simulink model "Gemelo_Digital_RT_5_8_sinc_dig_real"  (R2025a)
settings: Solver=ode4  StartTime=0.0  StopTime=15  FixedStep=0.002  RelTol=1e-3  EnableMultiTasking=on
PreLoadFcn:
  | d=fileparts(get_param('Gemelo_Digital_RT_5_8_sinc_dig_real','FileName')); while ~isempty(d)&&~isfile(fullfile(d,'setup_paths.m')), n=fileparts(d); if strcmp(n,d),break;end; d=n; end; if isfile(fullfile(d,'setup_paths.m')), addpath(d); setup_paths; end
  | setup_swingup_quanser; Ensamblaje_pendulo_furuta_multibody_v4_DataFile;
InitFcn:
  | setup_swingup_quanser; Ensamblaje_pendulo_furuta_multibody_v4_DataFile;
undefined symbols (not defined in the file): alpha, alpha_m, g, HIL, Jp_cm, Ksync_tau, kt, l, mp, mr, p, qc_get_step_size, r, Rm, theta, theta_m, Vm, x_m, xhat
libraries: fl_lib x7, nesl_utility x7, simulink x5, quarc_library x4, sm_lib x2, ee_lib x1
settings Model: ExtModeTrigDuration=10000  Creator=sebas  LastModifiedBy=sebas
settings SolverCC: AlgebraicLoopSolver=TrustRegion  PositivePriorityOrder=on
settings DataIOCC: ReturnWorkspaceOutputs=off
settings DebuggingCC: UnconnectedInputMsg=warning  UnconnectedOutputMsg=warning  UnconnectedLineMsg=warning  ArithmeticOperatorsInVariantConditions=warning
settings ModelReferenceCC: EnableRefExpFcnMdlSchedulingChecks=on
settings SFSimCC: SimUseLocalCustomCode=off  CustomCodeUndefinedFunction=UseInterfaceOnly
settings RTWCC: SystemTargetFile=quarc_win64.tlc  TemplateMakefile=quarc_default_tmf  RTWUseLocalCustomCode=off  Toolchain=QUARC win64 | nmake (64-bit Windows)  BuildConfiguration=Faster Runs  GPUComputeCapability=3.5  Description=QUARC Win64 Target Using Toolchain
settings CodeAppCC: StateflowObjectComments=on
settings STFCustomTargetCC: SystemTargetFile=quarc_win64.tlc  TargetLangStandard=C99 (ISO)  MultiwordLength=2048.0  DynamicStringBufferSize=256.0  ConcurrentExecutionCompliant=on  UseToolchainInfoCompliant=on
settings ConfigComp: CovMetricSettings=dswe

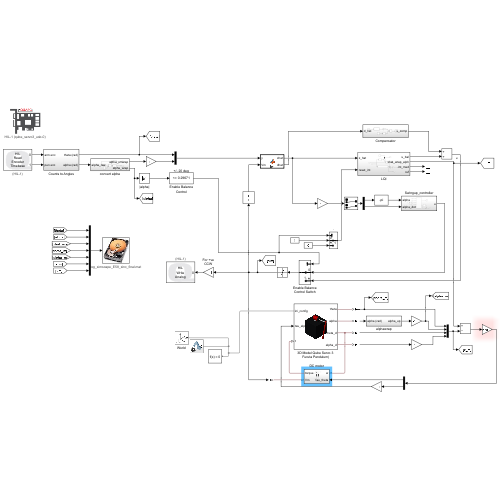
[thumbnail: Simulink's stored preview of the top-level diagram]
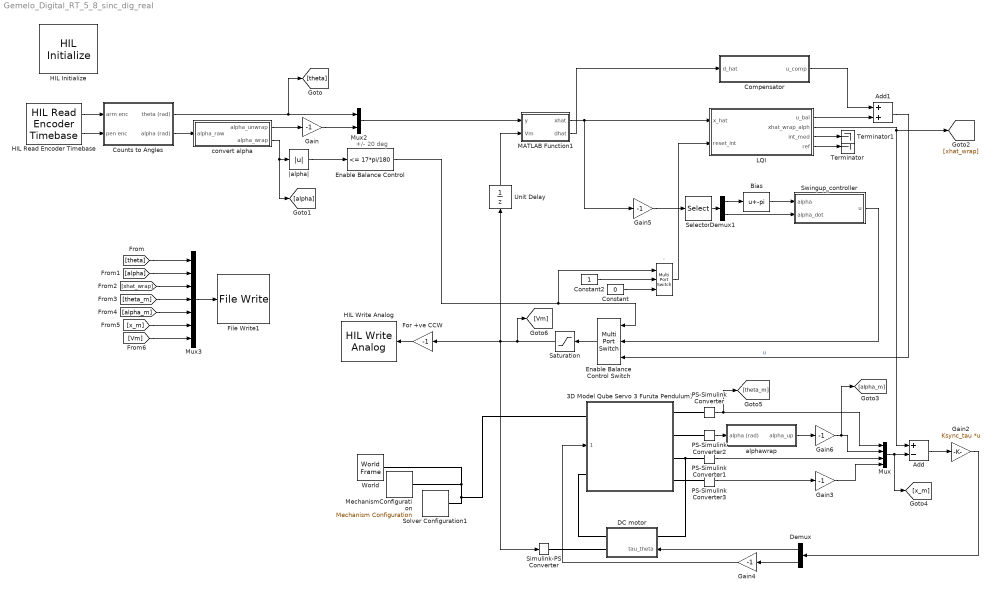
== system Gemelo_Digital_RT_5_8_sinc_dig_real ==
  note: +/- 20 deg
  . : MultiPortSwitch  DataPortOrder=Zero-based contiguous  Inputs=2  zeroidx=on  SaturateOnIntegerOverflow=off  InputSameDT=off
  3D Model Qube Servo 3 Furuta Pendulum) : Subsystem  ReferencedSubsystem=Model3d_Furuta_Pendulum
      settings: PortSchema="{\"entries\":[{\"content\":{\"sides\":[{\"content\":{\"connectorIds\":[\"LConn1\",\"In1\",\"RConn1\"]},\"type\":\"ConnectorPlacement.EquallySpacedRectSide\",\"uuid\":\"212e22e8-83aa-4288-bac8-5ec5012ee4e1\"},{\"content\":{\"connectorIds\":[\"RConn2\",\"RConn3\",\"RConn4\",\"RConn5\"],\"side\":\"RIGHT\"},\"type\":\"ConnectorPlacement.EquallySpacedRectSide\",\"uuid\":\"3ce73576-5c91-4b8f-99f3-bf7d5d6df258\"},{\"content\":{\"side\":\"TOP\"},\"type\":\"ConnectorPlacement.EquallySpacedRectSide\",\"uuid\":\"0c3f09e1-5576-45f6-bf17-671c1b7b7e25\"}]},\"type\":\"ConnectorPlacement.EquallySpacedConnector\",\"uuid\":\"8a7c1845-9713-4869-bdf4-33668feaed10\"}],\"packageUris\":[\"http://schema.mathworks.com/mf0/Connector/R2020b\"],\"version\":\"1.0\"}"
  Add : Sum  Inputs=+-
  Add1 : Sum
  Bias : Bias  Bias=-pi  SaturateOnIntegerOverflow=off
  Compensator : Subsystem
  Constant : Constant  Value=0
  Constant2 : Constant
  Counts to Angles : Subsystem
  DC motor : Subsystem
      settings: PortSchema="{\"entries\":[{\"content\":{\"sides\":[{\"content\":{\"connectorIds\":[\"LConn1\",\"In1\"]},\"type\":\"ConnectorPlacement.EquallySpacedRectSide\",\"uuid\":\"69bd88ca-8c2a-4f56-9568-a6ac34231cb3\"},{\"content\":{\"connectorIds\":[\"RConn1\",\"RConn2\"],\"side\":\"RIGHT\"},\"type\":\"ConnectorPlacement.EquallySpacedRectSide\",\"uuid\":\"19dd9353-83e6-4777-a984-67df33566e37\"},{\"content\":{\"side\":\"TOP\"},\"type\":\"ConnectorPlacement.EquallySpacedRectSide\",\"uuid\":\"45c5d2e2-678e-4947-ac23-f07febb6517c\"}]},\"type\":\"ConnectorPlacement.EquallySpacedConnector\",\"uuid\":\"c676389f-ef6f-4d18-b05a-27f295148147\"}],\"packageUris\":[\"http://schema.mathworks.com/mf0/Connector/R2020b\"],\"version\":\"1.0\"}"
  Demux : Demux  Outputs=2
  Demux1 : Demux  Outputs=2
  Enable Balance Control : simulink/Logic and Bit Operations/Compare To Constant  relop=<=  const=17*pi/180  OutDataTypeStr=boolean  ZeroCross=off
  Enable Balance Control Switch : MultiPortSwitch  DataPortOrder=Zero-based contiguous  Inputs=2  zeroidx=on  SaturateOnIntegerOverflow=off  InputSameDT=off
  File Write1 : quarc_library/Sinks/To Target/File Write  source=Specify via dialog (do not evaluate)  file_name=log_simscape_E58_sinc_final.mat  variable_name=theta,alpha,xhat,theta_m,alpha_m,x_m,Vm  decimation=1  sample_time=-1  file_format=MAT-file v.4  options=No header or footer  append=off  encoding=Default  bitrate=0
      settings: AttributesFormatString=%<file_name>  SourceProductName=QUARC Targets
  For +ve CCW : Gain  Gain=-1
  Gain{,3..6} (5 alike) : Gain  Gain=-1
  Gain2 : Gain  Gain=Ksync_tau  Multiplication=Matrix(K*u)
  HIL Initialize : quarc_library/Data Acquisition/Generic/Configuration/HIL Initialize  object_name=HIL-1  board_type=qube_servo3_usb  board_number=0  board_options=deadband_compensation=0.3;pwm_en=0;enc0_velocity=3.0;enc1_velocity=3.0;min_diode_compensation=0.3;max_diode_compensation=1.5;  exclusive=off  active=on  hardware_clocks=[0]  clock_modes=[]  initial_clock_frequencies=[]  set_clock_params_at_start=off  set_clock_params_at_switch_in=off  set_clock_frequencies_at_start=off  set_clock_frequencies_at_switch_in=off  analog_input_channels=[0]  analog_input_configurations=[]  analog_input_maximums=3  analog_input_minimums=-3  set_analog_input_params_at_start=off  set_analog_input_params_at_switch_in=off  analog_output_channels=[0]  analog_output_maximums=15  analog_output_minimums=-15  initial_analog_outputs=[0]  final_analog_outputs=[0]  watchdog_analog_outputs=0  set_analog_output_params_at_start=off  set_analog_output_params_at_switch_in=off  set_analog_outputs_at_start=on  set_analog_outputs_at_switch_in=off  set_analog_outputs_at_terminate=on  set_analog_outputs_at_switch_out=off  set_analog_outputs_on_watchdog=on  digital_input_channels=[]  digital_output_channels=[0]  digital_output_configuration=[]  initial_digital_outputs=[1]  final_digital_outputs=[0]  watchdog_digital_outputs=[0]  set_digital_output_params_at_start=off  set_digital_output_params_at_switch_in=off  set_digital_outputs_at_start=on  set_digital_outputs_at_switch_in=off  set_digital_outputs_at_terminate=on  set_digital_outputs_at_switch_out=off  set_digital_outputs_on_watchdog=on  encoder_channels=[0:1]  quadrature=[4]  encoder_filter_frequency=[]  initial_encoder_counts=[0]  set_encoder_params_at_start=off  set_encoder_params_at_switch_in=off  set_encoder_counts_at_start=on  set_encoder_counts_at_switch_in=off  pwm_channels=[]  pwm_modes=[0]  pwm_frequency=23195  pwm_configuration=[1]  pwm_alignment=[0]  pwm_polarity=[1]  pwm_leading_deadband=[0]  pwm_trailing_deadband=[0]  initial_pwm_outputs=[0]  final_pwm_outputs=[0]  watchdog_pwm_outputs=[]  set_pwm_params_at_start=off  set_pwm_params_at_switch_in=off  set_pwm_outputs_at_start=off  set_pwm_outputs_at_switch_in=off  set_pwm_outputs_at_terminate=off  set_pwm_outputs_at_switch_out=off  set_pwm_outputs_on_watchdog=off  other_output_channels=[11000:11002]  initial_other_outputs=[0 1 0]  final_other_outputs=[1 0 0]  watchdog_other_outputs=[0 0 1]  set_other_outputs_at_start=on  set_other_outputs_at_switch_in=off  set_other_outputs_at_terminate=on  set_other_outputs_at_switch_out=off  set_other_outputs_on_watchdog=on
  HIL Read Encoder Timebase : quarc_library/Data Acquisition/Generic/Timebases/HIL Read Encoder Timebase  object_name=HIL-1  clock=0  channels=[0:1]  active=on  vector_output=off  data_type_mode=Inherit via back propagation  data_type=double  overflow_mode=Error on overflow  samples_in_buffer=max(ceil(1/qc_get_step_size), 1)
  HIL Write Analog : quarc_library/Data Acquisition/Generic/Immediate I//O/HIL Write Analog  object_name=HIL-1  channels=[0]  sample_time=-1  active=off  vector_input=off
  LQI : Subsystem
  MATLAB Function1 : MATLAB Function  TreatAsAtomicUnit=on
  MechanismConfiguration : sm_lib/Utilities/Mechanism Configuration  UniformGravity=Constant  GravityVector=[0 -9.7807 0]  GravityVectorUnits=m/s^2  LinearizationDelta=0.001  JointModeTransitionNonlinearIterations=2
  Mux : Mux
  Mux2 : Mux  Inputs=2
  Mux3 : Mux  Inputs=7
  PS-Simulink Converter{,1..3} (4 alike) : nesl_utility/PS-Simulink Converter  PhysicalDomain=network_engine_domain  SubClassName=ps_output  LeftPortType=input  RightPortType=output  PseudoPeriodic=off  Frequencies=[]  VectorFormat=inherit  Unit=inherit  AffineConversion=off
  Saturation : Saturate  UpperLimit=10  LowerLimit=-10
  Selector : Selector  InputPortWidth=4  IndexOptions=Index vector (dialog)  Indices=[2 4]  OutputSizes=1
  Simulink-PS Converter : nesl_utility/Simulink-PS Converter  PhysicalDomain=network_engine_domain  SubClassName=ps_input  LeftPortType=input  RightPortType=output  PseudoPeriodic=off  Frequencies=[]  NoiseDistribution=none  NoiseParameters=[]  Unit=1  AffineConversion=off  FilteringAndDerivatives=filter  SimscapeFilterOrder=1  InputFilterTimeConstant=0.001  UdotUserProvided=0
  Solver Configuration1 : nesl_utility/Solver Configuration  PhysicalDomain=network_engine_domain  SubClassName=solver  LeftPortType=input  RightPortType=generic  Tones=[]  Harmonics=[]  SimulateNoise=off  Profile=off  UseLocalSampling=off  EnableSwitchedLinearOptims=on  FrequencyDomain=off  UseCCode=off  RelTol=0.001  AbsTol=0.001  MinStep=1e-09  ToWorkspace=off  RevertToSquareIcSolve=off  NumHomotopyIterations=100  PhasorMode=off  PhasorModeNumHarmonics=1  ConsistencySolver=NEWTON_XTOL_AFTER_FTOL  IndexReductionMethod=DerivativeReplacement  DoDC=off  ResidualTolerance=1e-09  ConsistencyTolSource=GLOBAL  ConsistencyAbsTol=0.001  ConsistencyRelTol=0.001  ConsistencyTolFactor=1e-9  UseLocalSolver=on  LocalSolverChoice=NE_BACKWARD_EULER_ADVANCER  ResolveIndetEquations=on  FunctionEvalNumThread=1  LocalSolverSampleTime=0.002  DoFixedCost=on  MaxNonlinIter=5  MaxModeIter=2  ComputeImpulses=on  ImpulseIterations=2  LinearAlgebra=auto  LinearAlgebraNumThread=0  EquationFormulation=NE_TIME_EF  DelaysMemoryBudget=1024  AutomaticFiltering=on  FilteringTimeConstant=0.001  PartitionStorageMethod=AS_NEEDED  PartitionMemoryBudget=1024  PartitionMethod=ROBUST  MultibodyUseLocalSolver=off  MultibodyLocalSolverChoice=ODE1  MultibodyLocalSolverSampleTime=0.002
  Swingup_controller : Subsystem
  Terminator : Terminator
  Terminator1 : Terminator
  Unit Delay : UnitDelay  SampleTime=-1  HasFrameUpgradeWarning=on
  World : sm_lib/Frames and Transforms/World Frame
  alphawrap : Subsystem
  convert alpha : Subsystem
  |alpha| : Abs  SaturateOnIntegerOverflow=off
  wires:
  Gain4/1 -> 3D Model Qube Servo 3 Furuta Pendulum)/1
  PS-Simulink Converter/1 -> [theta_m], Mux/1
  alphawrap/1(alpha_up) -> Gain6/1
  PS-Simulink Converter3/1 -> Gain3/1
  Gain3/1 -> Mux/4
  PS-Simulink Converter1/1 -> Mux/3
  Gain2/1 -> Demux/1
  LQI/2(xhat_wrap_alph) -> [xhat_wrap], Add/1
  Add/1 -> Gain2/1
  Demux/1 -> DC motor/1(tau_theta)
  Demux/2 -> Gain4/1
  Mux/1 -> [x_m], Add/2
  Counts to Angles/1(theta (rad)) -> [theta], Mux2/1
  HIL Read Encoder Timebase/2 -> Counts to Angles/2(pen enc)
  HIL Read Encoder Timebase/1 -> Counts to Angles/1(arm enc)
  Saturation/1 -> [Vm], Simulink-PS Converter/1, For +ve CCW/1, Unit Delay/1
  MATLAB Function1/2(dhat) -> Compensator/1(d_hat)
  Mux3/1 -> File Write1/1
  MATLAB Function1/1(xhat) -> Gain5/1, LQI/1(x_hat)
  Swingup_controller/1(u) -> Enable Balance Control Switch/2
  LQI/1(u_bal) -> Add1/2
  Constant/1 -> ./3
  Counts to Angles/2(alpha (rad)) -> convert alpha/1(alpha_raw)
  Add1/1 -> Enable Balance Control Switch/3  "u"
  Demux1/2 -> Swingup_controller/2(alpha_dot)
  Constant2/1 -> ./2
  convert alpha/2(alpha_wrap) -> [alpha], |alpha|/1
  Gain5/1 -> Selector/1
  Selector/1 -> Demux1/1
  |alpha|/1 -> Enable Balance Control/1
  Demux1/1 -> Bias/1
  ./1 -> LQI/2(reset_int)
  Enable Balance Control Switch/1 -> Saturation/1
  convert alpha/1(alpha_unwrap) -> Gain/1
  Enable Balance Control/1 -> Enable Balance Control Switch/1, ./1
  For +ve CCW/1 -> HIL Write Analog/1
  Mux2/1 -> MATLAB Function1/1(y)
  Bias/1 -> Swingup_controller/1(alpha)
  Unit Delay/1 -> MATLAB Function1/2(Vm)
  Compensator/1(u_comp) -> Add1/1
  PS-Simulink Converter2/1 -> alphawrap/1(alpha (rad))
  Gain/1 -> Mux2/2
  Gain6/1 -> [alpha_m], Mux/2
  LQI/4(ref) -> Terminator/1
  LQI/3(int_med) -> Terminator1/1
  [theta] -> Mux3/1
  [alpha] -> Mux3/2
  [xhat_wrap] -> Mux3/3
  [theta_m] -> Mux3/4
  [alpha_m] -> Mux3/5
  [x_m] -> Mux3/6
  [Vm] -> Mux3/7
  connections:
  World/RConn1 -- MechanismConfiguration/RConn1 -- Solver Configuration1/RConn1 -- 3D Model Qube Servo 3 Furuta Pendulum)/LConn1
  Simulink-PS Converter/RConn1 -- DC motor/RConn2
  3D Model Qube Servo 3 Furuta Pendulum)/RConn2 -- PS-Simulink Converter/LConn1
  3D Model Qube Servo 3 Furuta Pendulum)/RConn3 -- PS-Simulink Converter2/LConn1
  3D Model Qube Servo 3 Furuta Pendulum)/RConn4 -- DC motor/LConn1 -- PS-Simulink Converter1/LConn1
  3D Model Qube Servo 3 Furuta Pendulum)/RConn5 -- PS-Simulink Converter3/LConn1
  DC motor/RConn1 -- 3D Model Qube Servo 3 Furuta Pendulum)/RConn1

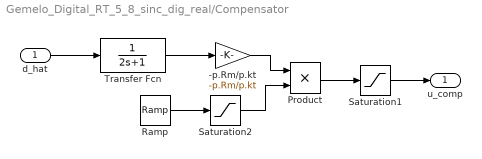
== system Gemelo_Digital_RT_5_8_sinc_dig_real/Compensator ==
  d_hat : Inport
  -p.Rm/p.kt : Gain  Gain=-p.Rm/p.kt
  Product : Product
  Ramp : simulink/Sources/Ramp  slope=0.5  start=0  InitialOutput=0
  Saturation1 : Saturate  UpperLimit=2  LowerLimit=-2
  Saturation2 : Saturate  UpperLimit=1  LowerLimit=0
  Transfer Fcn : TransferFcn  Denominator=[2 1]
  u_comp : Outport
  wires:
  Saturation1/1 -> u_comp/1
  Transfer Fcn/1 -> -p.Rm/p.kt/1
  -p.Rm/p.kt/1 -> Product/1
  Saturation2/1 -> Product/2
  Ramp/1 -> Saturation2/1
  d_hat/1 -> Transfer Fcn/1
  Product/1 -> Saturation1/1

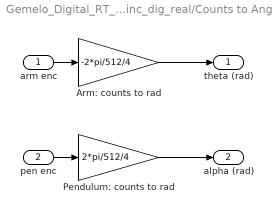
== system Gemelo_Digital_RT_5_8_sinc_dig_real/Counts to Angles ==
  arm enc : Inport
  pen enc : Inport  Port=2
  Arm: counts to rad : Gain  Gain=-2*pi/512/4
  Pendulum: counts to rad : Gain  Gain=2*pi/512/4
  theta (rad) : Outport  VectorParamsAs1DForOutWhenUnconnected=off
  alpha (rad) : Outport  Port=2  VectorParamsAs1DForOutWhenUnconnected=off
  wires:
  pen enc/1 -> Pendulum: counts to rad/1
  arm enc/1 -> Arm: counts to rad/1
  Arm: counts to rad/1 -> theta (rad)/1
  Pendulum: counts to rad/1 -> alpha (rad)/1

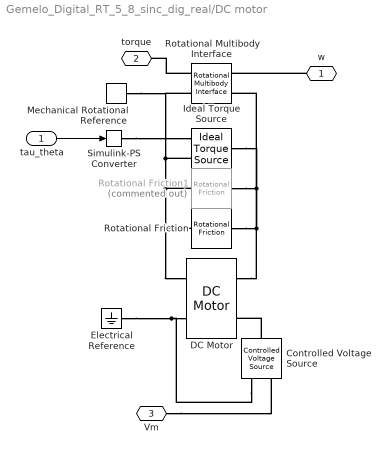
== system Gemelo_Digital_RT_5_8_sinc_dig_real/DC motor ==
  tau_theta : Inport
  Controlled Voltage Source : fl_lib/Electrical/Electrical Sources/Controlled Voltage Source
  DC Motor : ee_lib/Electromechanical/Brushed Motors/DC Motor  field_option=ee.enum.field_option.pm  Rf=100 Ohm  Lf=1 H  Laf=0.15 H  If0=0 A  parameterization=ee.enum.dcparam_option.circuit_param  Ra=7.5 Ohm  La=1.15e-3 H  emf_or_torque=ee.enum.emf_or_torque.kv  Kv=0.0422 V*s/rad  Ki=0.0422 N*m/A  T_stall=0.24e-3 N*m  w_max=5400 rpm  w_rated=4579 rpm  P_rated=9.8 W  V_rated=24 V  lam_param=ee.enum.lam_param.damping  i_noload=16 mA  V_i_noload=24 V  J=1.4e-6 kg*m^2  lam=1*4.8390e-6 N*m*s/rad  speed0=0 rpm  alpha=3.93e-3 1/K  Tmeas=25 degC  thermal_mass=100 J/K  initial_temperature=25 degC
  Electrical Reference : fl_lib/Electrical/Electrical Elements/Electrical Reference
  Ideal Torque Source : fl_lib/Mechanical/Mechanical Sources/Ideal Torque Source
  Mechanical Rotational Reference : fl_lib/Mechanical/Rotational Elements/Mechanical Rotational Reference
  Rotational Friction : fl_lib/Mechanical/Rotational Elements/Rotational Friction  brkwy_trq=1*2.910555e-05+1*4.081637e-05 N*m  brkwy_vel=1.082312e-02 rad/s  Col_trq=2.910555e-05 N*m  visc_coef=4.321929e-06 N*m*s/rad  w_specify=off  w_priority=None  w=0 rad/s  w_nominal_specify=off  w_nominal_value=1  w_nominal_unit=rad/s  t_specify=off  t_priority=None  t=0 N*m  t_nominal_specify=off  t_nominal_value=1  t_nominal_unit=N*m
  Rotational Friction1 : fl_lib/Mechanical/Rotational Elements/Rotational Friction  Commented=on  brkwy_trq=7.066e-04 N*m  brkwy_vel=0.1 rad/s  Col_trq=7.066e-09 N*m  visc_coef=0 N*m*s/rad  w_specify=off  w_priority=None  w=0 rad/s  w_nominal_specify=off  w_nominal_value=1  w_nominal_unit=rad/s  t_specify=off  t_priority=None  t=0 N*m  t_nominal_specify=off  t_nominal_value=1  t_nominal_unit=N*m
  Rotational Multibody Interface : fl_lib/Mechanical/Multibody Interfaces/Rotational Multibody Interface
  Simulink-PS Converter : nesl_utility/Simulink-PS Converter  PhysicalDomain=network_engine_domain  SubClassName=ps_input  LeftPortType=input  RightPortType=output  PseudoPeriodic=off  Frequencies=[]  NoiseDistribution=none  NoiseParameters=[]  Unit=1  AffineConversion=off  FilteringAndDerivatives=filter  SimscapeFilterOrder=1  InputFilterTimeConstant=0.001  UdotUserProvided=0
  w : PMIOPort  Side=Left
  torque : PMIOPort  Port=2  Side=Right
  Vm : PMIOPort  Port=3  Side=Right
  wires:
  tau_theta/1 -> Simulink-PS Converter/1
  connections:
  Rotational Friction/LConn1 -- Rotational Friction1/LConn1 -- Ideal Torque Source/LConn1 -- Rotational Multibody Interface/RConn2 -- DC Motor/LConn2
  Rotational Friction/RConn1 -- Ideal Torque Source/RConn2 -- Rotational Multibody Interface/LConn2 -- Mechanical Rotational Reference/LConn1 -- Rotational Friction1/RConn1 -- DC Motor/RConn2
  Vm/RConn1 -- Controlled Voltage Source/RConn1
  w/RConn1 -- Rotational Multibody Interface/RConn1
  DC Motor/RConn1 -- Electrical Reference/LConn1 -- Controlled Voltage Source/RConn2
  Controlled Voltage Source/LConn1 -- DC Motor/LConn1
  Rotational Multibody Interface/LConn1 -- torque/RConn1
  Simulink-PS Converter/RConn1 -- Ideal Torque Source/RConn1

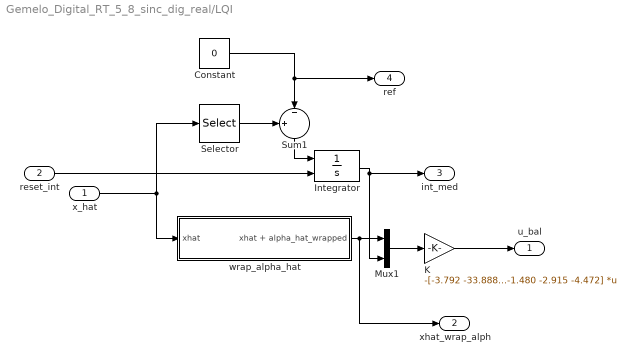
== system Gemelo_Digital_RT_5_8_sinc_dig_real/LQI ==
  x_hat : Inport
  reset_int : Inport  Port=2
  Constant : Constant  Value=0
  Integrator : Integrator  ExternalReset=level hold  LimitOutput=on  UpperSaturationLimit=2  LowerSaturationLimit=-2
  K : Gain  Gain=-[-3.792 -33.888 -1.480 -2.915 -4.472]  Multiplication=Matrix(K*u)
  Mux1 : Mux  Inputs=2
  Selector : Selector  InputPortWidth=4  IndexOptions=Index vector (dialog)  Indices=[1]  OutputSizes=1
  Sum1 : Sum  Inputs=+|-||
  wrap_alpha_hat : Subsystem
  u_bal : Outport
  xhat_wrap_alph : Outport  Port=2
  int_med : Outport  Port=3
  ref : Outport  Port=4
  wires:
  Integrator/1 -> int_med/1, Mux1/2
  Mux1/1 -> K/1
  Constant/1 -> ref/1, Sum1/2
  Sum1/1 -> Integrator/1
  Selector/1 -> Sum1/1
  K/1 -> u_bal/1
  reset_int/1 -> Integrator/2
  x_hat/1 -> wrap_alpha_hat/1(xhat), Selector/1
  wrap_alpha_hat/1(xhat + alpha_hat_wrapped) -> xhat_wrap_alph/1, Mux1/1

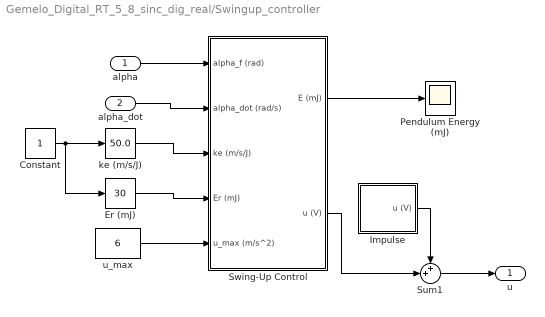
== system Gemelo_Digital_RT_5_8_sinc_dig_real/Swingup_controller ==
  alpha : Inport
  alpha_dot : Inport  Port=2
  Constant : Constant
  Er (mJ) : simulink/Math Operations/Slider Gain  gain=30  low=0  high=100
  Impulse : Subsystem
  Pendulum Energy (mJ) : Scope
      settings: ActiveDisplayYMinimum=-1.7076335355968837  ActiveDisplayYMaximum=4.1343640569805871  DataLoggingVariableName=ScopeData3
  Sum1 : Sum  Inputs=++|
  Swing-Up Control : Subsystem
  ke (m/s/J) : simulink/Math Operations/Slider Gain  gain=50.0  low=0  high=100
  u_max : Constant  Value=6
  u : Outport
  wires:
  alpha/1 -> Swing-Up Control/1(alpha_f (rad))
  Sum1/1 -> u/1
  u_max/1 -> Swing-Up Control/5(u_max (m/s^2))
  Impulse/1(u (V)) -> Sum1/1
  Swing-Up Control/1(E (mJ)) -> Pendulum Energy (mJ)/1
  Swing-Up Control/2(u (V)) -> Sum1/2
  ke (m/s/J)/1 -> Swing-Up Control/3(ke (m/s/J))
  Constant/1 -> Er (mJ)/1, ke (m/s/J)/1
  Er (mJ)/1 -> Swing-Up Control/4(Er (mJ))
  alpha_dot/1 -> Swing-Up Control/2(alpha_dot (rad/s))

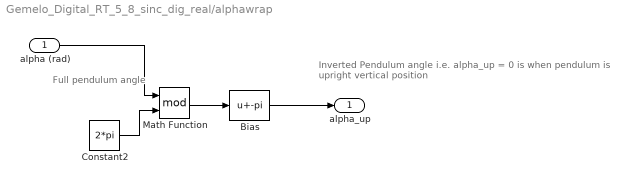
== system Gemelo_Digital_RT_5_8_sinc_dig_real/alphawrap ==
  note: Full pendulum angle
  note: Inverted Pendulum angle
      | i.e. alpha_up = 0 is when pendulum is upright vertical position
  alpha (rad) : Inport
  Bias : Bias  Bias=-pi  SaturateOnIntegerOverflow=off
  Constant2 : Constant  Value=2*pi
  Math Function : Math  Operator=mod  SignedPower=on
  alpha_up : Outport  VectorParamsAs1DForOutWhenUnconnected=off
  wires:
  Math Function/1 -> Bias/1
  Bias/1 -> alpha_up/1
  Constant2/1 -> Math Function/2
  alpha (rad)/1 -> Math Function/1

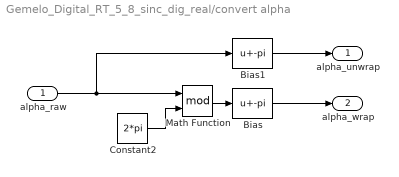
== system Gemelo_Digital_RT_5_8_sinc_dig_real/convert alpha ==
  alpha_raw : Inport
  Bias : Bias  Bias=-pi  SaturateOnIntegerOverflow=off
  Bias1 : Bias  Bias=-pi  SaturateOnIntegerOverflow=off
  Constant2 : Constant  Value=2*pi
  Math Function : Math  Operator=mod  SignedPower=on
  alpha_unwrap : Outport
  alpha_wrap : Outport  Port=2
  wires:
  Math Function/1 -> Bias/1
  Bias/1 -> alpha_wrap/1
  Constant2/1 -> Math Function/2
  alpha_raw/1 -> Bias1/1, Math Function/1
  Bias1/1 -> alpha_unwrap/1

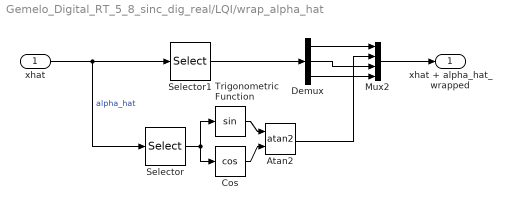
== system Gemelo_Digital_RT_5_8_sinc_dig_real/LQI/wrap_alpha_hat ==
  xhat : Inport
  Atan2 : Trigonometry  Operator=atan2
  Cos : Trigonometry  Operator=cos
  Demux : Demux  Outputs=3
  Mux2 : Mux
  Selector : Selector  InputPortWidth=4  IndexOptions=Index vector (dialog)  Indices=[2]  OutputSizes=1
  Selector1 : Selector  InputPortWidth=4  IndexOptions=Index vector (dialog)  Indices=[1 3 4]  OutputSizes=1
  Trigonometric Function : Trigonometry
  xhat + alpha_hat_wrapped : Outport
  wires:
  Selector/1 -> Cos/1, Trigonometric Function/1
  Mux2/1 -> xhat + alpha_hat_wrapped/1
  Cos/1 -> Atan2/2
  xhat/1 -> Selector/1, Selector1/1  "alpha_hat"
  Trigonometric Function/1 -> Atan2/1
  Demux/2 -> Mux2/3
  Selector1/1 -> Demux/1
  Demux/1 -> Mux2/1
  Demux/3 -> Mux2/4
  Atan2/1 -> Mux2/2

== system Gemelo_Digital_RT_5_8_sinc_dig_real/Swingup_controller/Impulse ==
  Impulse Amplitude : Gain  Gain=0.2
  Step : Step  SampleTime=0
  Step1 : Step  Time=1.1  After=-1  SampleTime=0
  Sum : Sum  Inputs=|++
  u (V) : Outport  VectorParamsAs1DForOutWhenUnconnected=off
  wires:
  Impulse Amplitude/1 -> u (V)/1
  Sum/1 -> Impulse Amplitude/1
  Step/1 -> Sum/1
  Step1/1 -> Sum/2

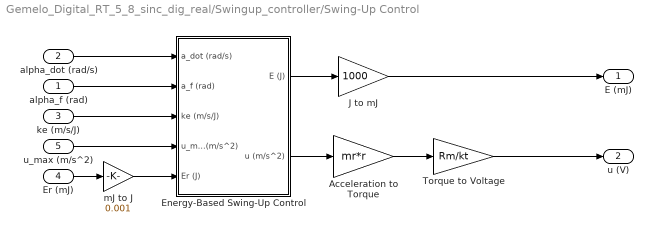
== system Gemelo_Digital_RT_5_8_sinc_dig_real/Swingup_controller/Swing-Up Control ==
  alpha_f (rad) : Inport
  alpha_dot (rad/s) : Inport  Port=2
  ke (m/s/J) : Inport  Port=3
  Er (mJ) : Inport  Port=4
  u_max (m/s^2) : Inport  Port=5
  Acceleration to Torque : Gain  Gain=mr*r
  Energy-Based Swing-Up Control : Subsystem
  J to mJ : Gain  Gain=1000
  Torque to Voltage : Gain  Gain=Rm/kt
  mJ to J : Gain  Gain=0.001
  E (mJ) : Outport  VectorParamsAs1DForOutWhenUnconnected=off
  u (V) : Outport  Port=2  VectorParamsAs1DForOutWhenUnconnected=off
  wires:
  mJ to J/1 -> Energy-Based Swing-Up Control/5(Er (J))
  alpha_dot (rad/s)/1 -> Energy-Based Swing-Up Control/1(a_dot (rad/s))
  Torque to Voltage/1 -> u (V)/1
  J to mJ/1 -> E (mJ)/1
  Er (mJ)/1 -> mJ to J/1
  Acceleration to Torque/1 -> Torque to Voltage/1
  u_max (m/s^2)/1 -> Energy-Based Swing-Up Control/4(u_max (m/s^2))
  ke (m/s/J)/1 -> Energy-Based Swing-Up Control/3(ke (m/s/J))
  alpha_f (rad)/1 -> Energy-Based Swing-Up Control/2(a_f (rad))
  Energy-Based Swing-Up Control/1(E (J)) -> J to mJ/1
  Energy-Based Swing-Up Control/2(u (m/s^2)) -> Acceleration to Torque/1

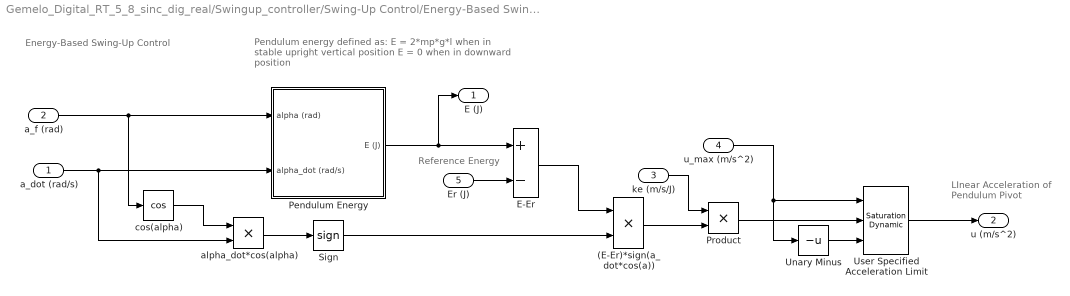
== system Gemelo_Digital_RT_5_8_sinc_dig_real/Swingup_controller/Swing-Up Control/Energy-Based Swing-Up Control ==
  note: Pendulum energy defined as:
      | E = 2*mp*g*l when in stable upright vertical position
      | E = 0 when in downward position
  note: Reference Energy
  note: LInear Acceleration of
      | Pendulum Pivot
  note: Energy-Based Swing-Up Control
  a_dot (rad/s) : Inport
  a_f (rad) : Inport  Port=2
  ke (m/s/J) : Inport  Port=3
  u_max (m/s^2) : Inport  Port=4
  Er (J) : Inport  Port=5
  (E-Er)*sign(a_dot*cos(a)) : Product  RndMeth=Zero
  E-Er : Sum  Inputs=+-
  Pendulum Energy : Subsystem
  Product : Product  RndMeth=Zero
  Sign : Signum
  Unary Minus : UnaryMinus
  User Specified Acceleration Limit : simulink/Discontinuities/Saturation Dynamic  OutMin=[]  OutMax=[]  OutDataTypeStr=Inherit: Same as second input  OutDataType=fixdt(1, 16)  OutScaling=2^-10  DoSatur=off
  alpha_dot*cos(alpha) : Product  RndMeth=Zero
  cos(alpha) : Trigonometry  Operator=cos
  E (J) : Outport  VectorParamsAs1DForOutWhenUnconnected=off
  u (m/s^2) : Outport  Port=2  VectorParamsAs1DForOutWhenUnconnected=off
  wires:
  User Specified Acceleration Limit/1 -> u (m/s^2)/1
  Unary Minus/1 -> User Specified Acceleration Limit/3
  u_max (m/s^2)/1 -> Unary Minus/1, User Specified Acceleration Limit/1
  Product/1 -> User Specified Acceleration Limit/2
  ke (m/s/J)/1 -> Product/1
  Er (J)/1 -> E-Er/2
  (E-Er)*sign(a_dot*cos(a))/1 -> Product/2
  a_dot (rad/s)/1 -> Pendulum Energy/2(alpha_dot (rad/s)), alpha_dot*cos(alpha)/2
  Pendulum Energy/1(E (J)) -> E-Er/1, E (J)/1
  E-Er/1 -> (E-Er)*sign(a_dot*cos(a))/1
  cos(alpha)/1 -> alpha_dot*cos(alpha)/1
  alpha_dot*cos(alpha)/1 -> Sign/1
  Sign/1 -> (E-Er)*sign(a_dot*cos(a))/2
  a_f (rad)/1 -> cos(alpha)/1, Pendulum Energy/1(alpha (rad))

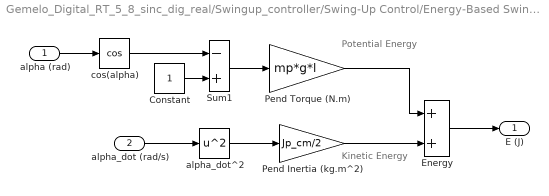
== system Gemelo_Digital_RT_5_8_sinc_dig_real/Swingup_controller/Swing-Up Control/Energy-Based Swing-Up Control/Pendulum Energy ==
  note: Potential Energy
  note: Kinetic Energy
  alpha (rad) : Inport
  alpha_dot (rad/s) : Inport  Port=2
  Constant : Constant
  Energy : Sum  SaturateOnIntegerOverflow=on
  Pend Inertia (kg.m^2) : Gain  Gain=Jp_cm/2
  Pend Torque (N.m) : Gain  Gain=mp*g*l
  Sum1 : Sum  Inputs=-+  SaturateOnIntegerOverflow=on
  alpha_dot^2 : Math  Operator=square  SignedPower=on
  cos(alpha) : Trigonometry  Operator=cos
  E (J) : Outport  VectorParamsAs1DForOutWhenUnconnected=off
  wires:
  cos(alpha)/1 -> Sum1/1
  Energy/1 -> E (J)/1
  alpha_dot (rad/s)/1 -> alpha_dot^2/1
  alpha (rad)/1 -> cos(alpha)/1
  Pend Torque (N.m)/1 -> Energy/1
  alpha_dot^2/1 -> Pend Inertia (kg.m^2)/1
  Pend Inertia (kg.m^2)/1 -> Energy/2
  Constant/1 -> Sum1/2
  Sum1/1 -> Pend Torque (N.m)/1

== matlab function Gemelo_Digital_RT_5_8_sinc_dig_real/MATLAB Function1 ==
  settings: updateMethod=DISCRETE  sampleTime=0.002
  data: y input; xhat output; Vm input; dhat output
function [xhat, dhat] = fcn(y, Vm)
   %#codegen
   [xhat, dhat] = ekf_step(y, Vm);
   end
